simulink model "VehCtrlMdel240926_2018b_amkspdlimit"  (R2019b)
settings: Solver=FixedStepDiscrete  StartTime=0.0  StopTime=20  FixedStep=0.0005  RelTol=1e-3  EnableMultiTasking=on
undefined symbols (not defined in the file): Ax_OffSet, Ay_OffSet, Caf, Car, DiscIntNeverNeededParam, dwf, dwr, h, i1, i2, I_AN06_5V, I_AN07_5V, I_AN08_5V, I_AN09_5V, I_SW01_L, I_SW03_L, Iz, Kc, Ki, Kp, Ldwf, Ldwr, lf, lr, m, O_SW12_HS1A, O_SW14_HS1A, Offset_Angle, PWM3, Qa, Ra, Rt, thr1, thr2, thr3, thr4, thr5, TrqRquRate, YawRate_OffSet
libraries: simulink x150, ec5744lib x122, canmsglib x18
(part 4 of 5)

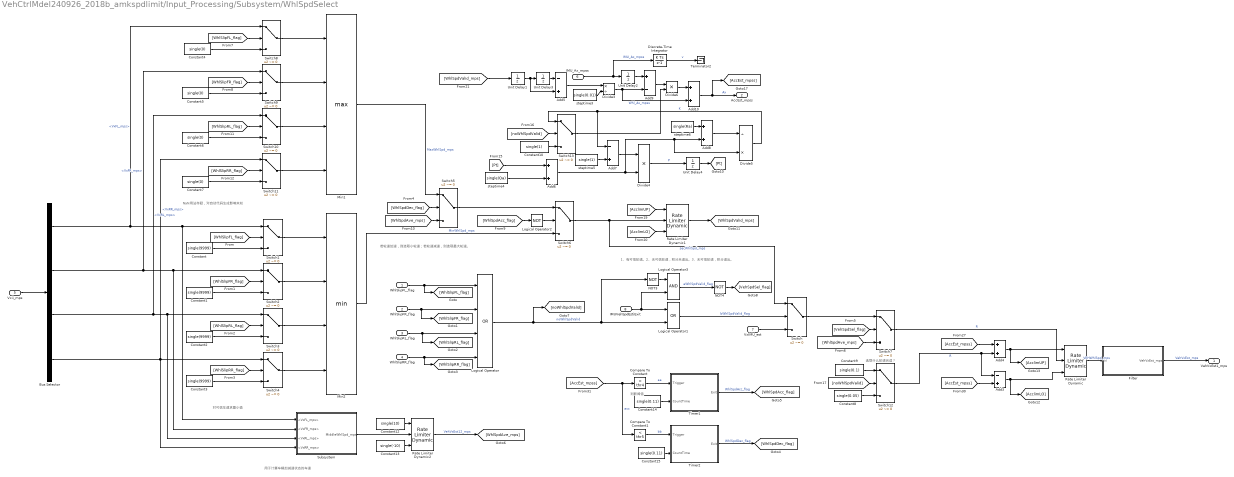
== system VehCtrlMdel240926_2018b_amkspdlimit/Input_Processing/Subsystem/WhlSpdSelect ==
  note: 用于计算车辆加减速状态的车速
  note: 1、有可信轮速。2、无可信轮速，积分未退出。3、无可信轮速，积分退出。
  note: 选取什么轮速合适？
  note: 判断阈值
  note: 若轮速加速，则选取小轮速；若轮速减速，则选取最大轮速。
  note: NaN用法存疑，对自动代码生成影响未知
  note: 对可信车速求最小值
  WhlSlipFL_flag : Inport
  WhlSlipFR_flag : Inport  Port=2
  WhlSlipRL_flag : Inport  Port=3
  WhlSlipRR_flag : Inport  Port=4
  Vxii_mps : Inport  Port=5
  IMU_Ax_mpss : Inport  Port=6
  VxIMU_est : Inport  Port=7
  IMUVehSpdEstiExit : Inport  Port=8
  Add{4,6,8,10} (4 alike) : Sum
  Add3 : Sum  Inputs=-+
  Add5 : Sum  Inputs=-+
  Add7 : Sum  Inputs=-+
  Add9 : Sum  Inputs=+-
  Bus Selector : BusSelector  OutputSignals=VxFL_mps,VxFR_mps,VxRL_mps,VxRR_mps
  Compare To Constant : simulink/Logic and Bit Operations/Compare To Constant  relop=>  const=thr4  OutDataTypeStr=boolean
  Compare To Constant1 : simulink/Logic and Bit Operations/Compare To Constant  relop=<  const=thr5  OutDataTypeStr=boolean
  Constant{,1..3} (4 alike) : Constant  Value=single(9999)
  Constant10 : Constant  Value=single(1)
  Constant12 : Constant  Value=single(10)
  Constant13 : Constant  Value=single(-10)
  Constant14 : Constant  Value=single(0.11)
  Constant15 : Constant  Value=single(0.11)
  Constant{4..7} (4 alike) : Constant  Value=single(0)
  Constant8 : Constant  Value=single(0.05)
  Constant9 : Constant  Value=single(0.1)
  Discrete-Time Integrator : DiscreteIntegrator  SampleTime=-1  ICPrevOutput=DiscIntNeverNeededParam  ICPrevScaledInput=DiscIntNeverNeededParam
  Divide3 : Product  Inputs=*/
  Divide4 : Product  Inputs=**
  Divide5 : Product  Inputs=/*
  Divide6 : Product  Inputs=**
  Filter : Subsystem
  Logical Operator : Logic  Operator=OR  Inputs=4  AllPortsSameDT=off  OutDataTypeStr=boolean
  Logical Operator1 : Logic  Operator=OR  AllPortsSameDT=off  OutDataTypeStr=boolean
  Logical Operator2 : Logic  Operator=NOT  AllPortsSameDT=off  OutDataTypeStr=boolean
  Logical Operator3 : Logic  AllPortsSameDT=off  OutDataTypeStr=boolean
  Min1 : MinMax  Function=max  Inputs=4
  Min2 : MinMax  Inputs=4
  NOT3 : Logic  Operator=NOT  AllPortsSameDT=off  OutDataTypeStr=boolean
  NOT4 : Logic  Operator=NOT  AllPortsSameDT=off  OutDataTypeStr=boolean
  Rate Limiter Dynamic : simulink/Discontinuities/Rate Limiter Dynamic
      settings: SourceProductName=Simulink
  Rate Limiter Dynamic1 : simulink/Discontinuities/Rate Limiter Dynamic
      settings: SourceProductName=Simulink
  Rate Limiter Dynamic2 : simulink/Discontinuities/Rate Limiter Dynamic
      settings: SourceProductName=Simulink
  Subsystem : Subsystem
  Switch{,1..13} (14 alike) : Switch  Criteria=u2 ~= 0
  Terminator2 : Terminator
  Timer1 : Stateflow chart  TreatAsAtomicUnit=on
  Timer2 : Stateflow chart  TreatAsAtomicUnit=on
  Unit Delay1 : UnitDelay  SampleTime=-1  HasFrameUpgradeWarning=on
  Unit Delay2 : UnitDelay  SampleTime=-1  HasFrameUpgradeWarning=on
  Unit Delay3 : UnitDelay  SampleTime=-1  HasFrameUpgradeWarning=on
  Unit Delay4 : UnitDelay  InitialCondition=0.01  SampleTime=-1  HasFrameUpgradeWarning=on
  steptime3 : Constant  Value=single(0.01)
  steptime4 : Constant  Value=single(Qa)
  steptime5 : Constant  Value=single(1)
  steptime6 : Constant  Value=single(Ra)
  VehVxEst1_mps : Outport
  AccEst_mpss : Outport  Port=2
  wires:
  Compare To Constant/1 -> Timer1/1(Trigger)  "aa"
  Vxii_mps/1 -> Bus Selector/1
  WhlSlipRR_flag/1 -> [WhlSlipRR_flag], Logical Operator/4
  Logical Operator3/1 -> NOT4/1  "aWhlSpdValid_flag"
  [VehSpdSel_flag] -> Switch7/2
  Logical Operator2/1 -> Switch6/2
  [WhlSlipFL_flag] -> Switch1/2
  Switch5/1 -> Switch6/1
  Constant/1 -> Switch1/3
  Compare To Constant1/1 -> Timer2/1(Trigger)  "bb"
  [WhlSpdAve_mps] -> Switch5/3
  Constant3/1 -> Switch4/3
  Logical Operator1/1 -> Switch/2  "bWhlSpdValid_flag"
  Switch4/1 -> Min2/4
  Constant2/1 -> Switch3/3
  [WhlSlipRR_flag] -> Switch4/2
  Switch1/1 -> Min2/1
  WhlSlipFR_flag/1 -> [WhlSlipFR_flag], Logical Operator/2
  [WhlSpdAcc_flag] -> Logical Operator2/1
  [WhlSlipRL_flag] -> Switch3/2
  Switch2/1 -> Min2/2
  WhlSlipFL_flag/1 -> [WhlSlipFL_flag], Logical Operator/1
  Constant1/1 -> Switch2/3
  [WhlSpdDec_flag] -> Switch5/2
  [WhlSlipFR_flag] -> Switch2/2
  WhlSlipRL_flag/1 -> [WhlSlipRL_flag], Logical Operator/3
  Switch3/1 -> Min2/3
  [WhlSpdAve_mps] -> Switch7/3
  Bus Selector/1 -> Switch8/1, Subsystem/1(<VxFL_mps>), Switch1/1  "<VxFL_mps>"
  Bus Selector/4 -> Subsystem/4(<VxRR_mps>), Switch11/1, Switch4/1  "<VxRR_mps>"
  [WhlSlipFR_flag] -> Switch9/2
  Bus Selector/2 -> Switch9/1, Subsystem/2(<VxFR_mps>), Switch2/1  "<VxFR_mps>"
  Constant5/1 -> Switch9/3
  Bus Selector/3 -> Switch10/1, Subsystem/3(<VxRL_mps>), Switch3/1  "<VxRL_mps>"
  [WhlSlipRL_flag] -> Switch10/2
  [WhlSlipRR_flag] -> Switch11/2
  Constant6/1 -> Switch10/3
  Constant7/1 -> Switch11/3
  Constant4/1 -> Switch8/3
  [WhlSlipFL_flag] -> Switch8/2
  Switch8/1 -> Min1/1
  Switch9/1 -> Min1/2
  Switch10/1 -> Min1/3
  Switch11/1 -> Min1/4
  Min1/1 -> Switch5/1  "MaxWhlSpd_mps"
  Subsystem/1(MiddleWhlSpd_mps) -> Rate Limiter Dynamic2/2
  Constant12/1 -> Rate Limiter Dynamic2/1
  Constant13/1 -> Rate Limiter Dynamic2/3
  Rate Limiter Dynamic2/1 -> [WhlSpdAve_mps]  "VehVxEst12_mps"
  Min2/1 -> Switch6/3  "MinWhlSpd_mps"
  IMUVehSpdEstiExit/1 -> Logical Operator3/2, Logical Operator1/1
  NOT3/1 -> Logical Operator3/1
  NOT4/1 -> [VehSpdSel_flag]
  Divide5/1 -> Add7/1, Switch13/1  "K"
  Unit Delay3/1 -> Add5/1
  steptime3/1 -> Divide3/2
  Add5/1 -> Divide3/1
  Unit Delay4/1 -> [Pt]
  [Pt] -> Add6/1
  steptime4/1 -> Add6/2
  Add6/1 -> Divide5/2, Add8/2, Divide4/2
  steptime5/1 -> Add7/2
  Add7/1 -> Divide4/1
  Divide4/1 -> Unit Delay4/1  "P"
  steptime6/1 -> Add8/1
  Add8/1 -> Divide5/1
  Divide3/1 -> Add10/2, Add9/2  "Whl_Ax_mpss"
  Add9/1 -> Divide6/1
  Divide6/1 -> Add10/1
  Add10/1 -> AccEst_mpss/1, [AccEst_mpss]  "Ax"
  IMU_Ax_mpss/1 -> Unit Delay2/1, Discrete-Time Integrator/1  "IMU_Ax_mpss"
  VxIMU_est/1 -> Switch/3
  Filter/1(VehVxEst_mps) -> VehVxEst1_mps/1  "VehVxEst_mps"
  Switch/1 -> Switch7/1
  Discrete-Time Integrator/1 -> Terminator2/1  "v"
  [AccEst_mpss] -> Add4/1
  [AccEst_mpss] -> Add3/2
  [WhlSpdValid_mps] -> Unit Delay1/1
  Unit Delay2/1 -> Add9/1
  Switch6/1 -> Switch/1, Rate Limiter Dynamic1/2  "secWhlSpd_mps"
  Add4/1 -> [AcclimUP], Rate Limiter Dynamic/1
  Add3/1 -> [AcclimLO], Rate Limiter Dynamic/3
  Switch7/1 -> Rate Limiter Dynamic/2  "R"
  Rate Limiter Dynamic/1 -> Filter/1(In)  "VEHWhlSpd_mps"
  Rate Limiter Dynamic1/1 -> [WhlSpdValid_mps]
  Unit Delay1/1 -> Add5/2, Unit Delay3/1
  [noWhlSpdValid] -> Switch12/2
  Constant8/1 -> Switch12/3
  Constant9/1 -> Switch12/1
  Switch12/1 -> Add3/1, Add4/2  "R"
  Switch13/1 -> Divide6/2
  [noWhlSpdValid] -> Switch13/2
  Constant10/1 -> Switch13/3
  [AcclimUP] -> Rate Limiter Dynamic1/1
  [AcclimLO] -> Rate Limiter Dynamic1/3
  Logical Operator/1 -> NOT3/1, Logical Operator1/2, [noWhlSpdValid]  "noWhlSpdValid"
  Timer1/1(Exit) -> [WhlSpdAcc_flag]  "WhlSpdAcc_flag"
  Constant14/1 -> Timer1/2(CountTime)
  Timer2/1(Exit) -> [WhlSpdDec_flag]  "WhlSpdDec_flag"
  Constant15/1 -> Timer2/2(CountTime)
  [AccEst_mpss] -> Compare To Constant1/1, Compare To Constant/1  "acc"

== system VehCtrlMdel240926_2018b_amkspdlimit/Input_Processing/Subsystem/坐标系转换 ==
  note: cos模块的单位是弧度制、
  note: 未考虑漂移工况
  note: 顺时针为正，逆时针为负。
  WhlSpdFL_mps : Inport
  WhlSpdFR_mps : Inport  Port=2
  WhlSpdRL_mps : Inport  Port=3
  WhlSpdRR_mps : Inport  Port=4
  IMU_YawRate_dps : Inport  Port=5
  WhlStrAngL_deg : Inport  Port=6
  WhlStrAngR_deg : Inport  Port=7
  Add : Sum  Inputs=+-
  Add1 : Sum
  Add2 : Sum  Inputs=+-
  Add3 : Sum
  Asin : Trigonometry  Operator=cos
  Asin1 : Trigonometry  Operator=cos
  Bus Creator : BusCreator  Inputs=4
  Constant : Constant  Value=single(Ldwr)
  Constant1 : Constant  Value=single(Ldwf)
  Gain : Gain  Gain=1/2
  Gain1 : Gain  Gain=1/2
  Gain2 : Gain  Gain=pi/180
  Gain3 : Gain  Gain=pi/180
  Gain4 : Gain  Gain=pi/180
  Product{,1..3} (4 alike) : Product
  Vxii_mps : Outport
  IMU_YawRate_dps1 : Outport  Port=2
  wires:
  Constant/1 -> Gain/1
  Gain/1 -> Product/2
  IMU_YawRate_dps/1 -> Gain4/1  "IMU_YawRate_dps"
  WhlSpdRL_mps/1 -> Add/1  "WhlSpdRL_mps"
  WhlSpdRR_mps/1 -> Add1/2  "WhlSpdRR_mps"
  Product/1 -> [Vldwr]
  [Vldwr] -> Add/2, Add1/1
  WhlSpdFL_mps/1 -> Product1/1  "WhlSpdFL_mps"
  WhlSpdFR_mps/1 -> Product2/2  "WhlSpdFR_mps"
  Constant1/1 -> Gain1/1
  Gain1/1 -> Product3/1
  Product3/1 -> [Vldwf]
  Product1/1 -> Add2/1  "1"
  [Vldwf] -> Add2/2, Add3/1  "3"
  Product2/1 -> Add3/2
  Add2/1 -> Bus Creator/1  "VxFL_mps"
  Add/1 -> Bus Creator/3  "VxRL_mps"
  Add3/1 -> Bus Creator/2  "VxFR_mps"
  Add1/1 -> Bus Creator/4  "VxRR_mps"
  Bus Creator/1 -> Vxii_mps/1
  Asin1/1 -> Product2/1
  WhlStrAngR_deg/1 -> Gain3/1  "WhlStrAngR_deg"
  WhlStrAngL_deg/1 -> Gain2/1  "WhlStrAngL_deg"
  Asin/1 -> Product1/2  "a"
  Gain2/1 -> Asin/1
  Gain3/1 -> Asin1/1
  Gain4/1 -> IMU_YawRate_dps1/1, Product/1, Product3/2

== system VehCtrlMdel240926_2018b_amkspdlimit/CTRL/MoTrqReq/TCS_PI+FF_Ctrl_FL/Latch_on ==
  Set : Inport
  Reset : Inport  Port=2
  Logical Operator4 : Logic  Operator=NOR  AllPortsSameDT=off  OutDataTypeStr=boolean
  Logical Operator5 : Logic  Operator=NOR  AllPortsSameDT=off  OutDataTypeStr=boolean
  Unit Delay1 : UnitDelay  SampleTime=-1  HasFrameUpgradeWarning=on
  flg_TCSActv : Outport
  wires:
  Logical Operator5/1 -> flg_TCSActv/1, Unit Delay1/1
  Reset/1 -> Logical Operator5/2
  Unit Delay1/1 -> Logical Operator4/1
  Set/1 -> Logical Operator4/2
  Logical Operator4/1 -> Logical Operator5/1

== system VehCtrlMdel240926_2018b_amkspdlimit/CTRL/MoTrqReq/TCS_PI+FF_Ctrl_FL/RisingTimer ==
  Set : Inport
  Timer : Inport  Port=2
  Add10 : Sum
  Min : MinMax  Inputs=2
  Relational Operator9 : RelationalOperator  OutDataTypeStr=boolean  RndMeth=Simplest
  Reset : Constant  Value=single(0)
  Steptime : Constant  Value=single(0.01)
  Switch6 : Switch  Criteria=u2 ~= 0
  Unit Delay1 : UnitDelay  SampleTime=-1  HasFrameUpgradeWarning=on
  TCSExit : Outport
  wires:
  Add10/1 -> Switch6/1
  Set/1 -> Switch6/2
  Min/1 -> Unit Delay1/1, Relational Operator9/1
  Unit Delay1/1 -> Add10/1
  Timer/1 -> Relational Operator9/2, Min/2
  Reset/1 -> Switch6/3
  Relational Operator9/1 -> TCSExit/1
  Steptime/1 -> Add10/2
  Switch6/1 -> Min/1

== system VehCtrlMdel240926_2018b_amkspdlimit/CTRL/MoTrqReq/TCS_PI+FF_Ctrl_FR/Latch_on ==
  Set : Inport
  Reset : Inport  Port=2
  Logical Operator4 : Logic  Operator=NOR  AllPortsSameDT=off  OutDataTypeStr=boolean
  Logical Operator5 : Logic  Operator=NOR  AllPortsSameDT=off  OutDataTypeStr=boolean
  Unit Delay1 : UnitDelay  SampleTime=-1  HasFrameUpgradeWarning=on
  flg_TCSActv : Outport
  wires:
  Logical Operator4/1 -> Logical Operator5/1
  Set/1 -> Logical Operator4/2
  Unit Delay1/1 -> Logical Operator4/1
  Reset/1 -> Logical Operator5/2
  Logical Operator5/1 -> Unit Delay1/1, flg_TCSActv/1

== system VehCtrlMdel240926_2018b_amkspdlimit/CTRL/MoTrqReq/TCS_PI+FF_Ctrl_FR/RisingTimer ==
  Set : Inport
  Timer : Inport  Port=2
  Add10 : Sum
  Min : MinMax  Inputs=2
  Relational Operator9 : RelationalOperator  OutDataTypeStr=boolean  RndMeth=Simplest
  Reset : Constant  Value=single(0)
  Steptime : Constant  Value=single(0.01)
  Switch6 : Switch  Criteria=u2 ~= 0
  Unit Delay1 : UnitDelay  SampleTime=-1  HasFrameUpgradeWarning=on
  TCSExit : Outport
  wires:
  Switch6/1 -> Min/1
  Steptime/1 -> Add10/2
  Relational Operator9/1 -> TCSExit/1
  Reset/1 -> Switch6/3
  Timer/1 -> Min/2, Relational Operator9/2
  Unit Delay1/1 -> Add10/1
  Min/1 -> Relational Operator9/1, Unit Delay1/1
  Set/1 -> Switch6/2
  Add10/1 -> Switch6/1

== system VehCtrlMdel240926_2018b_amkspdlimit/CTRL/MoTrqReq/TCS_PI+FF_Ctrl_R/Latch_on ==
  Set : Inport
  Reset : Inport  Port=2
  Logical Operator4 : Logic  Operator=NOR  AllPortsSameDT=off  OutDataTypeStr=boolean
  Logical Operator5 : Logic  Operator=NOR  AllPortsSameDT=off  OutDataTypeStr=boolean
  Unit Delay1 : UnitDelay  SampleTime=-1  HasFrameUpgradeWarning=on
  flg_TCSActv : Outport
  wires:
  Logical Operator5/1 -> flg_TCSActv/1, Unit Delay1/1
  Reset/1 -> Logical Operator5/2
  Unit Delay1/1 -> Logical Operator4/1
  Set/1 -> Logical Operator4/2
  Logical Operator4/1 -> Logical Operator5/1

== system VehCtrlMdel240926_2018b_amkspdlimit/CTRL/MoTrqReq/TCS_PI+FF_Ctrl_R/RisingTimer ==
  Set : Inport
  Timer : Inport  Port=2
  Add10 : Sum
  Min : MinMax  Inputs=2
  Relational Operator9 : RelationalOperator  OutDataTypeStr=boolean  RndMeth=Simplest
  Reset : Constant  Value=single(0)
  Steptime : Constant  Value=single(0.01)
  Switch6 : Switch  Criteria=u2 ~= 0
  Unit Delay1 : UnitDelay  SampleTime=-1  HasFrameUpgradeWarning=on
  TCSExit : Outport
  wires:
  Add10/1 -> Switch6/1
  Set/1 -> Switch6/2
  Min/1 -> Unit Delay1/1, Relational Operator9/1
  Unit Delay1/1 -> Add10/1
  Timer/1 -> Relational Operator9/2, Min/2
  Reset/1 -> Switch6/3
  Relational Operator9/1 -> TCSExit/1
  Steptime/1 -> Add10/2
  Switch6/1 -> Min/1

== system VehCtrlMdel240926_2018b_amkspdlimit/Input/ABS_Receive/ABS_BUS_state/IMU_state ==
  ID : Inport
  Msg : Inport  Port=2
  Enable : EnablePort
  CAN Unpack1 : canmsglib/CAN Unpack  CANdbFile=d:\Users\YJR\Desktop\DBC\Abs_Dev_Dbc_20240603_NingYuan.dbc  MsgList=ABS_Basic_Msg2  MsgName=ABS_Basic_Msg2  MsgIDType=Standard (11-bit identifier)  MsgIdentifier=1698  MsgLength=8  SignalInfo={'WS_FL','8','16','BE','signed','Standard','0','0.014063','0','-460.8','460.7859';'WS_FR','24','16','BE','signed','Standard','0','0.014063','0','-460.8','460.7859';'WS_RL','40','16','BE','signed','Standard','0','0.014063','0','-460.8','460.7859';'WS_RR','56','16','BE','signed','Standard','0','0.014063','0','-460.8','460.7859'}  IDPort=off  TimestampPort=off  ErrorPort=off  RemotePort=off  LengthPort=off  StatusPort=off  ApplyMinMax=off
      settings: SourceProductName=Simulink Real-Time  SourceProductBaseCode=XP  DataFormat=CANdb specified signals
  CANUnPackMessage4 : ec5744lib/RapidECU_U3/04CANCommunication/CANUnPackMessage  datalength=8  canmessagetype=Standard(11-bit ID)  sampletime=-1
      settings: SourceProductName=ECUCoder for MPC5744
  MeaModule1 : ec5744lib/RapidECU_U3/07Calibration/MeaModule  signal=ABS_WS_FR
      settings: SourceProductName=ECUCoder for MPC5744
  MeaModule2 : ec5744lib/RapidECU_U3/07Calibration/MeaModule  signal=ABS_WS_RL
      settings: SourceProductName=ECUCoder for MPC5744
  MeaModule3 : ec5744lib/RapidECU_U3/07Calibration/MeaModule  signal=ABS_WS_FL
      settings: SourceProductName=ECUCoder for MPC5744
  MeaModule4 : ec5744lib/RapidECU_U3/07Calibration/MeaModule  signal=ABS_WS_RR
      settings: SourceProductName=ECUCoder for MPC5744
  ABS_WS_FR : Outport  VectorParamsAs1DForOutWhenUnconnected=off
  ABS_WS_RL : Outport  Port=2  VectorParamsAs1DForOutWhenUnconnected=off
  ABS_WS_FL : Outport  Port=3  VectorParamsAs1DForOutWhenUnconnected=off
  ABS_WS_RR : Outport  Port=4  VectorParamsAs1DForOutWhenUnconnected=off
  wires:
  CAN Unpack1/3 -> MeaModule2/1  "ABS_WS_RL"
  CAN Unpack1/2 -> MeaModule1/1  "ABS_WS_FR"
  CAN Unpack1/1 -> MeaModule3/1  "ABS_WS_FL"
  CANUnPackMessage4/1 -> CAN Unpack1/1
  ID/1 -> CANUnPackMessage4/1
  Msg/1 -> CANUnPackMessage4/2
  CAN Unpack1/4 -> MeaModule4/1  "ABS_WS_RR"
  MeaModule3/1 -> ABS_WS_FL/1
  MeaModule1/1 -> ABS_WS_FR/1
  MeaModule2/1 -> ABS_WS_RL/1
  MeaModule4/1 -> ABS_WS_RR/1

== system VehCtrlMdel240926_2018b_amkspdlimit/Input/AMKMCU_Receive/FLAMKMCU/AMKMCU_state ==
  CANOK : Inport
  ID : Inport  Port=2
  Msg : Inport  Port=3
  function : TriggerPort  TriggerType=function-call  VariantControl=(inherit)
  MCU_state : Subsystem  TreatAsAtomicUnit=on
  FLAMKtoVCU1 : Outport  VectorParamsAs1DForOutWhenUnconnected=off
  wires:
  Msg/1 -> MCU_state/2(Msg)
  CANOK/1 -> MCU_state/Enable
  ID/1 -> MCU_state/1(ID)
  MCU_state/1(FLAMKMCUtoVCU1) -> FLAMKtoVCU1/1

== system VehCtrlMdel240926_2018b_amkspdlimit/Input/AMKMCU_Receive/FLAMKMCU/AMKMCU_state1 ==
  CANOK : Inport
  ID : Inport  Port=2
  Msg : Inport  Port=3
  function : TriggerPort  TriggerType=function-call  VariantControl=(inherit)
  Bus Creator : BusCreator  Inputs=2
  MCU_state : Subsystem  TreatAsAtomicUnit=on
  FLAMKMCUtoVCU2 : Outport  VectorParamsAs1DForOutWhenUnconnected=off
  wires:
  MCU_state/2(MCFL_ErrorInfo) -> Bus Creator/2
  MCU_state/1(MCFL_DiagnosticNum) -> Bus Creator/1
  Bus Creator/1 -> FLAMKMCUtoVCU2/1
  ID/1 -> MCU_state/1(ID)
  CANOK/1 -> MCU_state/Enable
  Msg/1 -> MCU_state/2(Msg)

== system VehCtrlMdel240926_2018b_amkspdlimit/Input/AMKMCU_Receive/FLAMKMCU/AMKMCU_state2 ==
  CANOK : Inport
  ID : Inport  Port=2
  Msg : Inport  Port=3
  function : TriggerPort  TriggerType=function-call  VariantControl=(inherit)
  Bus Creator : BusCreator  Inputs=3
  MCU_state : Subsystem  TreatAsAtomicUnit=on
  FLAMKMCUtoVCU3 : Outport  VectorParamsAs1DForOutWhenUnconnected=off
  wires:
  Msg/1 -> MCU_state/2(Msg)
  CANOK/1 -> MCU_state/Enable
  ID/1 -> MCU_state/1(ID)
  Bus Creator/1 -> FLAMKMCUtoVCU3/1  "Bus Creator"
  MCU_state/1(MCFL_TempIGBT) -> Bus Creator/1
  MCU_state/2(MCFL_TempInverter) -> Bus Creator/2
  MCU_state/3(MCFL_TempMotor) -> Bus Creator/3

== system VehCtrlMdel240926_2018b_amkspdlimit/Input/AMKMCU_Receive/FRAMKMCU/AMKMCU_state ==
  CANOK : Inport
  ID : Inport  Port=2
  Msg : Inport  Port=3
  function : TriggerPort  TriggerType=function-call  VariantControl=(inherit)
  Bus Creator : BusCreator  Inputs=12
  MCU_state : Subsystem  TreatAsAtomicUnit=on
  FRAMKMCUtoVCU1 : Outport  VectorParamsAs1DForOutWhenUnconnected=off
  wires:
  ID/1 -> MCU_state/1(ID)
  CANOK/1 -> MCU_state/Enable
  Msg/1 -> MCU_state/2(Msg)
  MCU_state/1(MCFR_ActualTorque) -> Bus Creator/1
  MCU_state/2(MCFR_ActualVelocity) -> Bus Creator/2
  MCU_state/3(MCFR_DCVoltage) -> Bus Creator/3
  MCU_state/4(MCFR_bDCOn) -> Bus Creator/4
  MCU_state/5(MCFR_bDerating) -> Bus Creator/5
  MCU_state/6(MCFR_bError) -> Bus Creator/6
  MCU_state/7(MCFR_bInverterOn) -> Bus Creator/7
  MCU_state/8(MCFR_bQuitDCOn) -> Bus Creator/8
  MCU_state/9(MCFR_bQuitInverterOn) -> Bus Creator/9
  MCU_state/10(MCFR_bReserve) -> Bus Creator/10
  MCU_state/11(MCFR_bSystemReady) -> Bus Creator/11
  MCU_state/12(MCFR_bWarn) -> Bus Creator/12
  Bus Creator/1 -> FRAMKMCUtoVCU1/1

== system VehCtrlMdel240926_2018b_amkspdlimit/Input/AMKMCU_Receive/FRAMKMCU/AMKMCU_state1 ==
  CANOK : Inport
  ID : Inport  Port=2
  Msg : Inport  Port=3
  function : TriggerPort  TriggerType=function-call  VariantControl=(inherit)
  Bus Creator : BusCreator  Inputs=2
  MCU_state : Subsystem  TreatAsAtomicUnit=on
  FRAMKMCUtoVCU2 : Outport  VectorParamsAs1DForOutWhenUnconnected=off
  wires:
  Msg/1 -> MCU_state/2(Msg)
  CANOK/1 -> MCU_state/Enable
  ID/1 -> MCU_state/1(ID)
  Bus Creator/1 -> FRAMKMCUtoVCU2/1
  MCU_state/1(MCFR_DiagnosticNum) -> Bus Creator/1
  MCU_state/2(MCFR_ErrorInfo) -> Bus Creator/2

== system VehCtrlMdel240926_2018b_amkspdlimit/Input/AMKMCU_Receive/FRAMKMCU/AMKMCU_state2 ==
  CANOK : Inport
  ID : Inport  Port=2
  Msg : Inport  Port=3
  function : TriggerPort  TriggerType=function-call  VariantControl=(inherit)
  Bus Creator : BusCreator  Inputs=3
  MCU_state : Subsystem  TreatAsAtomicUnit=on
  FRAMKMCUtoVCU3 : Outport  VectorParamsAs1DForOutWhenUnconnected=off
  wires:
  Bus Creator/1 -> FRAMKMCUtoVCU3/1
  ID/1 -> MCU_state/1(ID)
  CANOK/1 -> MCU_state/Enable
  Msg/1 -> MCU_state/2(Msg)
  MCU_state/1(MCFR_TempIGBT) -> Bus Creator/1
  MCU_state/2(MCFR_TempInverter) -> Bus Creator/2
  MCU_state/3(MCFR_TempMotor) -> Bus Creator/3

== system VehCtrlMdel240926_2018b_amkspdlimit/Input/BMS_Recive/ABS_BUS_state/IMU_state ==
  ID : Inport
  Msg : Inport  Port=2
  Enable : EnablePort
  CAN Unpack1 : canmsglib/CAN Unpack  CANdbFile=d:\Users\YJR\Desktop\DBC\bms.dbc  MsgList=BMS_HCU_INFO  MsgName=BMS_HCU_INFO  MsgIDType=Extended (29-bit identifier)  MsgIdentifier=408961267  MsgLength=8  SignalInfo={'BatAlmlv','52','4','LE','signed','Standard','0','1','0','0','4';'BatLife','56','8','LE','signed','Standard','0','1','0','0','255';'BatState','48','4','LE','signed','Standard','0','1','0','0','7';'LSBAz','24','8','LE','signed','Standard','0','0.1','-1000','-1012.8','-987.3';'LSBVz','8','8','LE','unsigned','Standard','0','0.1','0','0','9000';'MSBAz','16','8','LE','unsigned','Standard','0','0.1','-1000','-1000','-974.5';'MSBVz','0','8','LE','unsigned','Standard','0','0.1','0','0','9000';'SOCz','32','8','LE','signed','Standard','0','1','0','0','100';'SOHz','40','8','LE','signed','Standard','0','1','0','0','100'}  IDPort=off  TimestampPort=off  ErrorPort=off  RemotePort=off  LengthPort=off  StatusPort=off  ApplyMinMax=off
      settings: SourceProductName=Simulink Real-Time  SourceProductBaseCode=XP  DataFormat=CANdb specified signals
  CANUnPackMessage4 : ec5744lib/RapidECU_U3/04CANCommunication/CANUnPackMessage  datalength=8  canmessagetype=Extended(29-bit ID)  sampletime=-1
      settings: SourceProductName=ECUCoder for MPC5744
  BatAlmlv : Outport  VectorParamsAs1DForOutWhenUnconnected=off
  BatLife : Outport  Port=2  VectorParamsAs1DForOutWhenUnconnected=off
  BatState : Outport  Port=3  VectorParamsAs1DForOutWhenUnconnected=off
  LSBAz : Outport  Port=4  VectorParamsAs1DForOutWhenUnconnected=off
  LSBVz : Outport  Port=5  VectorParamsAs1DForOutWhenUnconnected=off
  MSBAz : Outport  Port=6  VectorParamsAs1DForOutWhenUnconnected=off
  MSBVz : Outport  Port=7  VectorParamsAs1DForOutWhenUnconnected=off
  SOCz : Outport  Port=8  VectorParamsAs1DForOutWhenUnconnected=off
  SOHz : Outport  Port=9  VectorParamsAs1DForOutWhenUnconnected=off
  wires:
  CANUnPackMessage4/1 -> CAN Unpack1/1
  ID/1 -> CANUnPackMessage4/1
  Msg/1 -> CANUnPackMessage4/2
  CAN Unpack1/1 -> BatAlmlv/1  "BatAlmlv"
  CAN Unpack1/2 -> BatLife/1  "BatLife"
  CAN Unpack1/3 -> BatState/1  "BatState"
  CAN Unpack1/4 -> LSBAz/1  "LSBAz"
  CAN Unpack1/5 -> LSBVz/1  "LSBVz"
  CAN Unpack1/6 -> MSBAz/1  "MSBAz"
  CAN Unpack1/7 -> MSBVz/1  "MSBVz"
  CAN Unpack1/8 -> SOCz/1  "SOCz"
  CAN Unpack1/9 -> SOHz/1  "SOHz"

== system VehCtrlMdel240926_2018b_amkspdlimit/Input/EMRAXMCU_RECIEVE/MCU_pwr/MCU_VCUMeter1 ==
  ID : Inport
  Msg : Inport  Port=2
  Enable : EnablePort
  CAN Unpack : canmsglib/CAN Unpack  CANdbFile=E:\candbc\MCU_No1.dbc  MsgList=(none)  MsgName=MCU2VCU2_ID1  MsgIDType=Extended (29-bit identifier)  MsgIdentifier=218089455  MsgLength=8  SignalInfo={'MCU2VCU2_Current_AC_Feedback_ID1','48','16','LE','unsigned','Standard','0','1.000000e-01','-1600','-1600','1600';'MCU2VCU2_Current_DC_feedback_ID1','32','16','LE','unsigned','Standard','0','1.000000e-01','-1600','-1600','1600';'MCU2VCU2_MCU_Temp_ID1','0','8','LE','unsigned','Standard','0','1','-50','-50','200';'MCU2VCU2_Motor_Temp_ID1','8','8','LE','unsigned','Standard','0','1','-50','-50','200';'MCU2VCU2_Voltage_Feedback_ID1','16','16','LE','unsigned','Standard','0','1.000000e-01','0','0','1000'}  IDPort=off  TimestampPort=off  ErrorPort=off  RemotePort=off  LengthPort=off  StatusPort=off  ApplyMinMax=off
      settings: SourceProductName=Vehicle Network Toolbox  SourceProductBaseCode=VN  DataFormat=CANdb specified signals
  CANUnPackMessage4 : ec5744lib/RapidECU_U3/04CANCommunication/CANUnPackMessage  datalength=8  canmessagetype=Extended(29-bit ID)  sampletime=-1
      settings: SourceProductName=ECUCoder for MPC5744
  MeaModule1 : ec5744lib/RapidECU_U3/07Calibration/MeaModule  signal=AC_current
      settings: SourceProductName=ECUCoder for MPC5744
  MeaModule2 : ec5744lib/RapidECU_U3/07Calibration/MeaModule  signal=DC_current
      settings: SourceProductName=ECUCoder for MPC5744
  MeaModule3 : ec5744lib/RapidECU_U3/07Calibration/MeaModule  signal=MCU_Temp
      settings: SourceProductName=ECUCoder for MPC5744
  MeaModule4 : ec5744lib/RapidECU_U3/07Calibration/MeaModule  signal=motor_Temp
      settings: SourceProductName=ECUCoder for MPC5744
  MeaModule5 : ec5744lib/RapidECU_U3/07Calibration/MeaModule  signal=voltage
      settings: SourceProductName=ECUCoder for MPC5744
  "AC_current " : Outport
  MCU_temp : Outport  Port=2
  current : Outport  Port=3
  motor_temp : Outport  Port=4
  voltage : Outport  Port=5
  wires:
  Msg/1 -> CANUnPackMessage4/2
  ID/1 -> CANUnPackMessage4/1
  CANUnPackMessage4/1 -> CAN Unpack/1
  CAN Unpack/1 -> MeaModule1/1  "AC_current"
  CAN Unpack/5 -> MeaModule5/1  "voltage"
  CAN Unpack/4 -> MeaModule4/1  "moter_temp"
  MeaModule1/1 -> "AC_current "/1
  MeaModule2/1 -> current/1
  CAN Unpack/3 -> MeaModule3/1  "MCU_temp"
  CAN Unpack/2 -> MeaModule2/1  "DC_current"
  MeaModule3/1 -> MCU_temp/1
  MeaModule4/1 -> motor_temp/1
  MeaModule5/1 -> voltage/1

== system VehCtrlMdel240926_2018b_amkspdlimit/Input/EMRAXMCU_RECIEVE/MCU_state/MCU_state ==
  ID : Inport
  Msg : Inport  Port=2
  Enable : EnablePort
  CAN Unpack : canmsglib/CAN Unpack  CANdbFile=E:\candbc\MCU_No1.dbc  MsgList=(none)  MsgName=MCU2VCU1_ID1  MsgIDType=Extended (29-bit identifier)  MsgIdentifier=218089199  MsgLength=8  SignalInfo={'MCU2VCU1_12V_error_ID1','45','1','LE','unsigned','Standard','0','1','0','0','1';'MCU2VCU1_Error_All_ID1','56','2','LE','unsigned','Standard','0','1','0','0','3';'MCU2VCU1_LowVoltage_error_ID1','46','1','LE','unsigned','Standard','0','1','0','0','1';'MCU2VCU1_MCU_Ready_ID1','40','1','LE','unsigned','Standard','0','1','0','0','1';'MCU2VCU1_MCU_Temp_error_ID1','48','1','LE','unsigned','Standard','0','1','0','0','1';'MCU2VCU1_Mode_Feedback_ID1','32','8','LE','unsigned','Standard','0','1','0','0','255';'MCU2VCU1_MotorTemp_error_ID1','49','1','LE','unsigned','Standard','0','1','0','0','1';'MCU2VCU1_OverCurrent_error_ID1','43','1','LE','unsigned','Standard','0','1','0','0','1';'MCU2VCU1_OverPower_error_ID1','47','1','LE','unsigned','Standard','0','1','0','0','1';'MCU2VCU1_OverVoltage_error_ID1','44','1','LE','unsigned','Standard','0','1','0','0','1';'MCU2VCU1_PrechargeState_ID1','41','1','LE','unsigned','Standard','0','1','0','0','1';'MCU2VCU1_Reslove_Error_ID1','42','1','LE','unsigned','Standard','0','1','0','0','1';'MCU2VCU1_Selfcheck_ID1','55','1','LE','unsigned','Standard','0','1','0','0','1';'MCU2VCU1_Speed_Feedback_ID1','0','16','LE','unsigned','Standard','0','5.000000e-01','-10000','-10000','10000';'MCU2VCU1_Torque_Feedback_ID1','16','16','LE','unsigned','Standard','0','1','0','0','1000'}  IDPort=off  TimestampPort=off  ErrorPort=off  RemotePort=off  LengthPort=off  StatusPort=off  ApplyMinMax=off
      settings: SourceProductName=Vehicle Network Toolbox  SourceProductBaseCode=VN  DataFormat=CANdb specified signals
  CANUnPackMessage4 : ec5744lib/RapidECU_U3/04CANCommunication/CANUnPackMessage  datalength=8  canmessagetype=Extended(29-bit ID)  sampletime=-1
      settings: SourceProductName=ECUCoder for MPC5744
  MeaModule : ec5744lib/RapidECU_U3/07Calibration/MeaModule  signal=RPM
      settings: SourceProductName=ECUCoder for MPC5744
  MeaModule1 : ec5744lib/RapidECU_U3/07Calibration/MeaModule  signal=alarm
      settings: SourceProductName=ECUCoder for MPC5744
  MeaModule2 : ec5744lib/RapidECU_U3/07Calibration/MeaModule  signal=L12V_error
      settings: SourceProductName=ECUCoder for MPC5744
  MeaModule3 : ec5744lib/RapidECU_U3/07Calibration/MeaModule  signal=controller_ready
      settings: SourceProductName=ECUCoder for MPC5744
  MeaModule5 : ec5744lib/RapidECU_U3/07Calibration/MeaModule  signal=selfcheck
      settings: SourceProductName=ECUCoder for MPC5744
  MeaModule6 : ec5744lib/RapidECU_U3/07Calibration/MeaModule  signal=trq
      settings: SourceProductName=ECUCoder for MPC5744
  12V_error : Outport
  alarm : Outport  Port=2
  undervol : Outport  Port=3
  controller_ready : Outport  Port=4
  MCU_temp_warn : Outport  Port=5
  mode_cmd8 : Outport  Port=6
  motor_temp_warn : Outport  Port=7
  overcur : Outport  Port=8
  pow_lim_warn : Outport  Port=9
  overvol : Outport  Port=10
  precharge : Outport  Port=11
  rotation_warn : Outport  Port=12
  selfcech : Outport  Port=13
  RPM : Outport  Port=14
  torque : Outport  Port=15
  wires:
  Msg/1 -> CANUnPackMessage4/2
  ID/1 -> CANUnPackMessage4/1
  CANUnPackMessage4/1 -> CAN Unpack/1
  MeaModule/1 -> RPM/1  "RPM"
  MeaModule1/1 -> alarm/1
  MeaModule2/1 -> 12V_error/1
  MeaModule3/1 -> controller_ready/1
  MeaModule5/1 -> selfcech/1
  MeaModule6/1 -> torque/1  "Trq"
  CAN Unpack/14 -> MeaModule/1  "RPM"
  CAN Unpack/15 -> MeaModule6/1  "Trq"
  CAN Unpack/13 -> MeaModule5/1
  CAN Unpack/11 -> precharge/1  "Precharge"
  CAN Unpack/10 -> overvol/1  "overvol"
  CAN Unpack/9 -> pow_lim_warn/1  "overpower"
  CAN Unpack/8 -> overcur/1  "overCurrent"
  CAN Unpack/7 -> motor_temp_warn/1  "motorTemp_error"
  CAN Unpack/6 -> mode_cmd8/1  "Mode"
  CAN Unpack/5 -> MCU_temp_warn/1  "MCU_Temp_error"
  CAN Unpack/4 -> MeaModule3/1  "MCU_Ready"
  CAN Unpack/3 -> undervol/1  "low_VOL"
  CAN Unpack/2 -> MeaModule1/1  "Error_ALL"
  CAN Unpack/1 -> MeaModule2/1  "12V_error"
  CAN Unpack/12 -> rotation_warn/1  "Reslove_error"

== system VehCtrlMdel240926_2018b_amkspdlimit/Input/IMU_Recieve/IMU_state/MCU_state ==
  ID : Inport
  Msg : Inport  Port=2
  Enable : EnablePort
  CAN Unpack : canmsglib/CAN Unpack  CANdbFile=d:\Users\YJR\Desktop\IMU.dbc  MsgList=(none)  MsgName=IMU  MsgIDType=Standard (11-bit identifier)  MsgIdentifier=513  MsgLength=8  SignalInfo={'IMU_Ax_Valid','1','1','LE','unsigned','Standard','0','1','0','-Inf','Inf';'IMU_Ax_Value','40','16','LE','unsigned','Standard','0','1.500000e-04','-4.915200e+00','-Inf','Inf';'IMU_Ay_Valid','2','1','LE','unsigned','Standard','0','1','0','-Inf','Inf';'IMU_Ay_Value','24','16','LE','unsigned','Standard','0','1.500000e-04','-4.915200e+00','-Inf','Inf';'IMU_DTC','4','4','LE','unsigned','Standard','0','1','0','-Inf','Inf';'IMU_Yaw_Valid','3','1','LE','unsigned','Standard','0','1','0','-Inf','Inf';'IMU_Yaw_Value','8','16','LE','unsigned','Standard','0','5.710000e-03','-1.872400e+02','-Inf','Inf'}  IDPort=off  TimestampPort=off  ErrorPort=off  RemotePort=off  LengthPort=off  StatusPort=off  ApplyMinMax=off
      settings: SourceProductName=Simulink Real-Time  SourceProductBaseCode=XP  DataFormat=CANdb specified signals
  CANUnPackMessage4 : ec5744lib/RapidECU_U3/04CANCommunication/CANUnPackMessage  datalength=8  canmessagetype=Standard(11-bit ID)  sampletime=-1
      settings: SourceProductName=ECUCoder for MPC5744
  MeaModule2 : ec5744lib/RapidECU_U3/07Calibration/MeaModule  signal=IMU_Ay_Value
      settings: SourceProductName=ECUCoder for MPC5744
  MeaModule3 : ec5744lib/RapidECU_U3/07Calibration/MeaModule  signal=IMU_Yaw_Value
      settings: SourceProductName=ECUCoder for MPC5744
  MeaModule4 : ec5744lib/RapidECU_U3/07Calibration/MeaModule  signal=IMU_Ax_Value
      settings: SourceProductName=ECUCoder for MPC5744
  IMU_Ax_Value : Outport  VectorParamsAs1DForOutWhenUnconnected=off
  IMU_Ay_Value : Outport  Port=2  VectorParamsAs1DForOutWhenUnconnected=off
  IMU_Yaw_Value : Outport  Port=3  VectorParamsAs1DForOutWhenUnconnected=off
  IMU_Ay_Valid : Outport  Port=4  VectorParamsAs1DForOutWhenUnconnected=off
  IMU_DTC : Outport  Port=5  VectorParamsAs1DForOutWhenUnconnected=off
  IMU_Yaw_Valid : Outport  Port=6  VectorParamsAs1DForOutWhenUnconnected=off
  IMU_Ax_Valid : Outport  Port=7  VectorParamsAs1DForOutWhenUnconnected=off
  wires:
  Msg/1 -> CANUnPackMessage4/2
  ID/1 -> CANUnPackMessage4/1
  CANUnPackMessage4/1 -> CAN Unpack/1
  CAN Unpack/2 -> MeaModule2/1
  CAN Unpack/3 -> IMU_Ay_Valid/1
  CAN Unpack/4 -> MeaModule4/1
  CAN Unpack/5 -> IMU_DTC/1
  CAN Unpack/7 -> MeaModule3/1
  CAN Unpack/6 -> IMU_Yaw_Valid/1
  CAN Unpack/1 -> IMU_Ax_Valid/1
  MeaModule2/1 -> IMU_Ax_Value/1
  MeaModule3/1 -> IMU_Yaw_Value/1
  MeaModule4/1 -> IMU_Ay_Value/1

== system VehCtrlMdel240926_2018b_amkspdlimit/Input/StrSnis_Receive/StrWhSnis_state/IMU_state ==
  ID : Inport
  Msg : Inport  Port=2
  Enable : EnablePort
  CAN Unpack : canmsglib/CAN Unpack  Commented=on  CANdbFile=d:\Users\YJR\Desktop\DBC\SWAS_3.dbc  MsgList=(none)  MsgName=PPEI_Steering_Wheel_Angle  MsgIDType=Standard (11-bit identifier)  MsgIdentifier=330  MsgLength=8  SignalInfo={'SAS_CheckSum','36','4','LE','unsigned','Standard','0','1','0','-Inf','Inf';'SAS_MassageCounter','32','4','LE','unsigned','Standard','0','1','0','0','15';'SAS_TrimmingFlag','26','1','LE','unsigned','Standard','0','1','0','0','255';'StrWhAng','8','16','BE','unsigned','Standard','0','1','0','0','65535';'StrWhAngV','16','8','LE','unsigned','Standard','0','1','0','0','1';'StrWhlAngSenCalFlag','25','1','LE','unsigned','Standard','0','1','0','0','3';'StrngWhlAngSnsrFailFlag','24','1','LE','unsigned','Standard','0','1','0','0','1'}  IDPort=off  TimestampPort=off  ErrorPort=off  RemotePort=off  LengthPort=off  StatusPort=off  ApplyMinMax=off
      settings: SourceProductName=Simulink Real-Time  SourceProductBaseCode=XP  DataFormat=CANdb specified signals
  CAN Unpack1 : canmsglib/CAN Unpack  CANdbFile=d:\Users\YJR\Desktop\DBC\SWAS.dbc  MsgList=PPEI_Steering_Wheel_Angle  MsgName=PPEI_Steering_Wheel_Angle  MsgIDType=Standard (11-bit identifier)  MsgIdentifier=330  MsgLength=8  SignalInfo={'StWhlAngAliveRollCnt','0','8','BE','unsigned','Standard','0','1','0','0','63';'StrWhAng','32','16','BE','unsigned','Standard','0','0.1','-779.3','-779.3','5774.2';'StrWhAngV','16','8','BE','unsigned','Standard','0','1','0','0','255'}  IDPort=off  TimestampPort=off  ErrorPort=off  RemotePort=off  LengthPort=off  StatusPort=off  ApplyMinMax=off
      settings: SourceProductName=Simulink Real-Time  SourceProductBaseCode=XP  DataFormat=CANdb specified signals
  CANUnPackMessage4 : ec5744lib/RapidECU_U3/04CANCommunication/CANUnPackMessage  datalength=8  canmessagetype=Standard(11-bit ID)  sampletime=-1
      settings: SourceProductName=ECUCoder for MPC5744
  MeaModule1 : ec5744lib/RapidECU_U3/07Calibration/MeaModule  signal=StrWhlAngAliveRollCnt
      settings: SourceProductName=ECUCoder for MPC5744
  MeaModule2 : ec5744lib/RapidECU_U3/07Calibration/MeaModule  signal=StrWhlAng
      settings: SourceProductName=ECUCoder for MPC5744
  MeaModule3 : ec5744lib/RapidECU_U3/07Calibration/MeaModule  signal=StrWhlAngV
      settings: SourceProductName=ECUCoder for MPC5744
  StrWhlAng : Outport  VectorParamsAs1DForOutWhenUnconnected=off
  StrWhlAngV : Outport  Port=2  VectorParamsAs1DForOutWhenUnconnected=off
  StrWhlAngAliveRollCnt : Outport  Port=3  VectorParamsAs1DForOutWhenUnconnected=off
  wires:
  Msg/1 -> CANUnPackMessage4/2
  ID/1 -> CANUnPackMessage4/1
  CANUnPackMessage4/1 -> CAN Unpack1/1
  CAN Unpack1/1 -> MeaModule1/1
  CAN Unpack1/2 -> MeaModule2/1
  CAN Unpack1/3 -> MeaModule3/1
  MeaModule1/1 -> StrWhlAngAliveRollCnt/1
  MeaModule2/1 -> StrWhlAng/1
  MeaModule3/1 -> StrWhlAngV/1

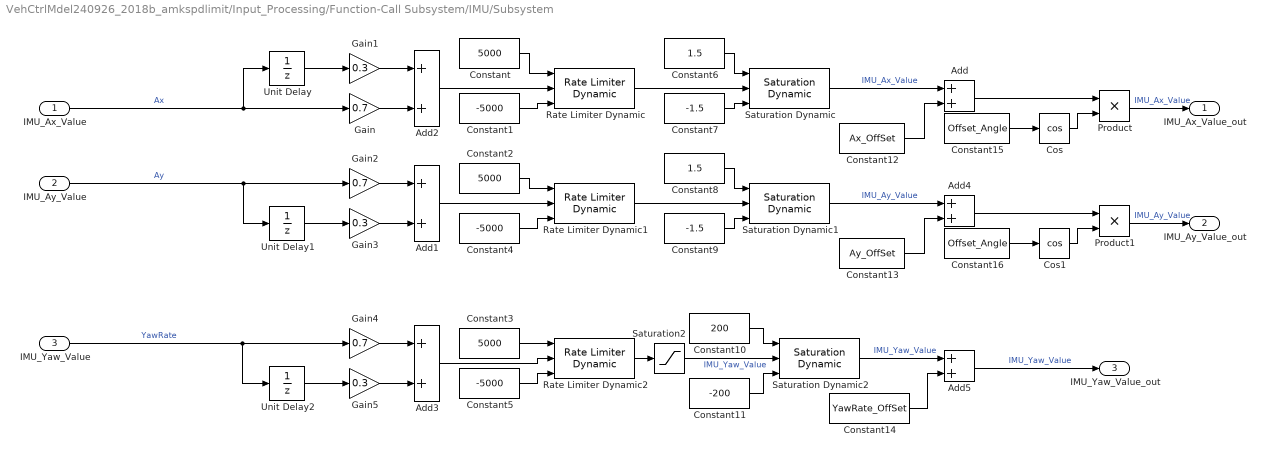
== system VehCtrlMdel240926_2018b_amkspdlimit/Input_Processing/Function-Call Subsystem/IMU/Subsystem ==
  IMU_Ax_Value : Inport
  IMU_Ay_Value : Inport  Port=2
  IMU_Yaw_Value : Inport  Port=3
  Add{,1..5} (6 alike) : Sum
  Constant : Constant  Value=5000
  Constant1 : Constant  Value=-5000
  Constant10 : Constant  Value=200  SampleTime=-1
  Constant11 : Constant  Value=-200  SampleTime=-1
  Constant12 : Constant  Value=Ax_OffSet
  Constant13 : Constant  Value=Ay_OffSet
  Constant14 : Constant  Value=YawRate_OffSet
  Constant15 : Constant  Value=Offset_Angle
  Constant16 : Constant  Value=Offset_Angle
  Constant2 : Constant  Value=5000
  Constant3 : Constant  Value=5000
  Constant4 : Constant  Value=-5000
  Constant5 : Constant  Value=-5000
  Constant6 : Constant  Value=1.5  SampleTime=-1
  Constant7 : Constant  Value=-1.5  SampleTime=-1
  Constant8 : Constant  Value=1.5  SampleTime=-1
  Constant9 : Constant  Value=-1.5  SampleTime=-1
  Cos : Trigonometry  Operator=cos
  Cos1 : Trigonometry  Operator=cos
  Gain : Gain  Gain=0.7
  Gain1 : Gain  Gain=0.3
  Gain2 : Gain  Gain=0.7
  Gain3 : Gain  Gain=0.3
  Gain4 : Gain  Gain=0.7
  Gain5 : Gain  Gain=0.3
  Product : Product
  Product1 : Product
  Rate Limiter Dynamic : simulink/Discontinuities/Rate Limiter Dynamic
      settings: SourceProductName=Simulink
  Rate Limiter Dynamic1 : simulink/Discontinuities/Rate Limiter Dynamic
      settings: SourceProductName=Simulink
  Rate Limiter Dynamic2 : simulink/Discontinuities/Rate Limiter Dynamic
      settings: SourceProductName=Simulink
  Saturation Dynamic : simulink/Discontinuities/Saturation Dynamic  OutMin=[]  OutMax=[]  OutDataTypeStr=Inherit: Same as second input  OutDataType=fixdt(1, 16)  OutScaling=2^-10  DoSatur=off
  Saturation Dynamic1 : simulink/Discontinuities/Saturation Dynamic  OutMin=[]  OutMax=[]  OutDataTypeStr=Inherit: Same as second input  OutDataType=fixdt(1, 16)  OutScaling=2^-10  DoSatur=off
  Saturation Dynamic2 : simulink/Discontinuities/Saturation Dynamic  OutMin=[]  OutMax=[]  OutDataTypeStr=Inherit: Same as second input  OutDataType=fixdt(1, 16)  OutScaling=2^-10  DoSatur=off
  Saturation2 : Saturate  UpperLimit=180  LowerLimit=-180
  Unit Delay : UnitDelay  SampleTime=-1  HasFrameUpgradeWarning=on
  Unit Delay1 : UnitDelay  SampleTime=-1  HasFrameUpgradeWarning=on
  Unit Delay2 : UnitDelay  SampleTime=-1  HasFrameUpgradeWarning=on
  IMU_Ax_Value_out : Outport  VectorParamsAs1DForOutWhenUnconnected=off
  IMU_Ay_Value_out : Outport  Port=2  VectorParamsAs1DForOutWhenUnconnected=off
  IMU_Yaw_Value_out : Outport  Port=3  VectorParamsAs1DForOutWhenUnconnected=off
  wires:
  IMU_Ay_Value/1 -> Unit Delay1/1, Gain2/1  "Ay"
  Unit Delay/1 -> Gain1/1
  Gain/1 -> Add2/2
  Constant2/1 -> Rate Limiter Dynamic1/1
  Constant/1 -> Rate Limiter Dynamic/1
  Add2/1 -> Rate Limiter Dynamic/2
  Gain2/1 -> Add1/1
  IMU_Yaw_Value/1 -> Gain4/1, Unit Delay2/1  "YawRate"
  Gain1/1 -> Add2/1
  Gain5/1 -> Add3/2
  IMU_Ax_Value/1 -> Gain/1, Unit Delay/1  "Ax"
  Constant11/1 -> Saturation Dynamic2/3
  Add1/1 -> Rate Limiter Dynamic1/2
  Unit Delay1/1 -> Gain3/1
  Constant8/1 -> Saturation Dynamic1/1
  Add3/1 -> Rate Limiter Dynamic2/2
  Constant4/1 -> Rate Limiter Dynamic1/3
  Rate Limiter Dynamic1/1 -> Saturation Dynamic1/2
  Constant1/1 -> Rate Limiter Dynamic/3
  Gain4/1 -> Add3/1
  Constant7/1 -> Saturation Dynamic/3
  Constant3/1 -> Rate Limiter Dynamic2/1
  Product/1 -> IMU_Ax_Value_out/1  "IMU_Ax_Value"
  Constant9/1 -> Saturation Dynamic1/3
  Add5/1 -> IMU_Yaw_Value_out/1  "IMU_Yaw_Value"
  Rate Limiter Dynamic2/1 -> Saturation2/1
  Saturation2/1 -> Saturation Dynamic2/2  "IMU_Yaw_Value"
  Constant10/1 -> Saturation Dynamic2/1
  Constant5/1 -> Rate Limiter Dynamic2/3
  Rate Limiter Dynamic/1 -> Saturation Dynamic/2
  Gain3/1 -> Add1/2
  Product1/1 -> IMU_Ay_Value_out/1  "IMU_Ay_Value"
  Constant6/1 -> Saturation Dynamic/1
  Unit Delay2/1 -> Gain5/1
  Saturation Dynamic/1 -> Add/1  "IMU_Ax_Value"
  Constant12/1 -> Add/2
  Saturation Dynamic1/1 -> Add4/1  "IMU_Ay_Value"
  Constant13/1 -> Add4/2
  Saturation Dynamic2/1 -> Add5/1  "IMU_Yaw_Value"
  Constant14/1 -> Add5/2
  Add/1 -> Product/1
  Cos/1 -> Product/2
  Constant15/1 -> Cos/1
  Constant16/1 -> Cos1/1
  Cos1/1 -> Product1/2
  Add4/1 -> Product1/1

== system VehCtrlMdel240926_2018b_amkspdlimit/Input_Processing/Subsystem/WhlSlpageJudgment/加速度差判断 ==
  note: 输出“1”代表判定有效
  <VxFL_mps> : Inport
  <VxFR_mps> : Inport  Port=2
  <VxRL_mps> : Inport  Port=3
  <VxRR_mps> : Inport  Port=4
  IMU_Ax_mpss : Inport  Port=5
  Abs{,1..3} (4 alike) : Abs
  Add{,1..3} (4 alike) : Sum  Inputs=+-
  Add{4..7} (4 alike) : Sum  Inputs=-+
  Compare To Constant{,1..3} (4 alike) : simulink/Logic and Bit Operations/Compare To Constant  relop=<=  const=thr2  OutDataTypeStr=boolean
  Divide{,1..3} (4 alike) : Product  Inputs=*/
  Filter : Subsystem
  Filter1 : Subsystem
  Filter2 : Subsystem
  Filter3 : Subsystem
  Unit Delay{,1..3} (4 alike) : UnitDelay  SampleTime=-1  HasFrameUpgradeWarning=on
  steptime{,1..3} (4 alike) : Constant  Value=single(0.01)
  y : Outport
  y1 : Outport  Port=2
  y2 : Outport  Port=3
  y3 : Outport  Port=4
  wires:
  Compare To Constant/1 -> y/1
  Compare To Constant2/1 -> y2/1
  Abs2/1 -> Compare To Constant2/1
  Add1/1 -> Abs1/1
  Abs/1 -> Compare To Constant/1
  [IMU_Ax_mpss] -> Add3/2
  [IMU_Ax_mpss] -> Add2/2
  [IMU_Ax_mpss] -> Add/2
  Abs3/1 -> Compare To Constant3/1
  Compare To Constant3/1 -> y3/1
  Compare To Constant1/1 -> y1/1
  [IMU_Ax_mpss] -> Add1/2
  Add/1 -> Abs/1
  Add3/1 -> Abs3/1
  Abs1/1 -> Compare To Constant1/1
  Add2/1 -> Abs2/1
  <VxFL_mps>/1 -> Add4/2, Unit Delay/1
  Unit Delay/1 -> Add4/1
  Add4/1 -> Divide/1
  steptime/1 -> Divide/2
  Divide/1 -> Filter/1(In)
  IMU_Ax_mpss/1 -> [IMU_Ax_mpss]
  steptime1/1 -> Divide1/2
  Add5/1 -> Divide1/1
  Unit Delay1/1 -> Add5/1
  <VxFR_mps>/1 -> Unit Delay1/1, Add5/2
  Divide1/1 -> Filter1/1(In)
  steptime2/1 -> Divide2/2
  Add6/1 -> Divide2/1
  Unit Delay2/1 -> Add6/1
  <VxRL_mps>/1 -> Unit Delay2/1, Add6/2
  Divide2/1 -> Filter2/1(In)
  steptime3/1 -> Divide3/2
  Add7/1 -> Divide3/1
  Unit Delay3/1 -> Add7/1
  <VxRR_mps>/1 -> Unit Delay3/1, Add7/2
  Divide3/1 -> Filter3/1(In)
  Filter/1(Out) -> Add/1
  Filter1/1(Out) -> Add1/1
  Filter2/1(Out) -> Add2/1
  Filter3/1(Out) -> Add3/1

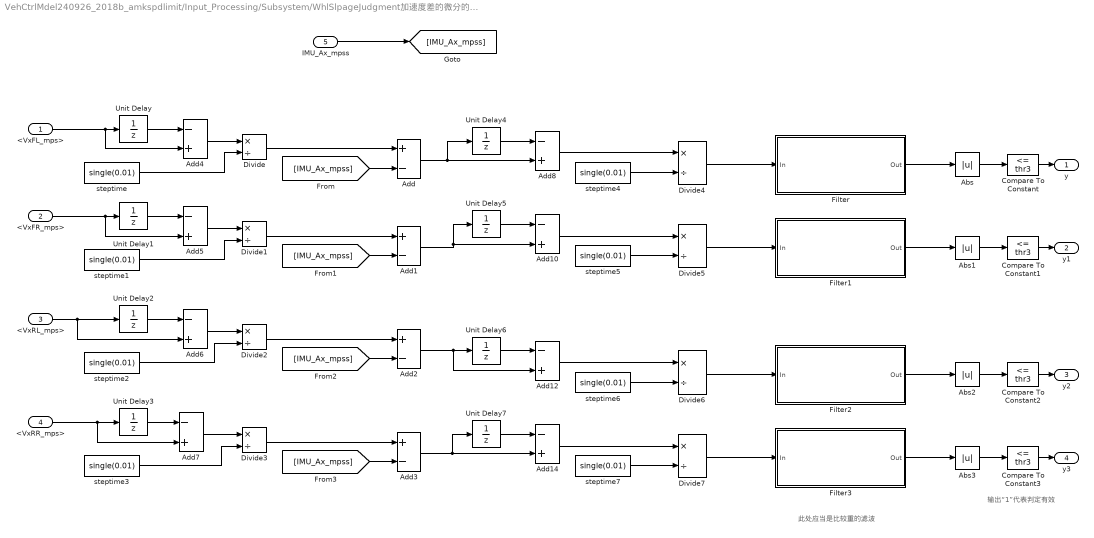
== system VehCtrlMdel240926_2018b_amkspdlimit/Input_Processing/Subsystem/WhlSlpageJudgment/加速度差的微分的判断 ==
  note: 此处应当是比较重的滤波
  note: 输出“1”代表判定有效
  <VxFL_mps> : Inport
  <VxFR_mps> : Inport  Port=2
  <VxRL_mps> : Inport  Port=3
  <VxRR_mps> : Inport  Port=4
  IMU_Ax_mpss : Inport  Port=5
  Abs{,1..3} (4 alike) : Abs
  Add{,1..3} (4 alike) : Sum  Inputs=+-
  Add{4..8,10,12,14} (8 alike) : Sum  Inputs=-+
  Compare To Constant{,1..3} (4 alike) : simulink/Logic and Bit Operations/Compare To Constant  relop=<=  const=thr3  OutDataTypeStr=boolean
  Divide{,1..7} (8 alike) : Product  Inputs=*/
  Filter : Subsystem
  Filter1 : Subsystem
  Filter2 : Subsystem
  Filter3 : Subsystem
  Unit Delay{,1..7} (8 alike) : UnitDelay  SampleTime=-1  HasFrameUpgradeWarning=on
  steptime{,1..7} (8 alike) : Constant  Value=single(0.01)
  y : Outport
  y1 : Outport  Port=2
  y2 : Outport  Port=3
  y3 : Outport  Port=4
  wires:
  Divide3/1 -> Add3/1
  <VxRR_mps>/1 -> Add7/2, Unit Delay3/1
  Unit Delay3/1 -> Add7/1
  Add7/1 -> Divide3/1
  steptime3/1 -> Divide3/2
  Divide2/1 -> Add2/1
  <VxRL_mps>/1 -> Add6/2, Unit Delay2/1
  Unit Delay2/1 -> Add6/1
  Add6/1 -> Divide2/1
  steptime2/1 -> Divide2/2
  Divide1/1 -> Add1/1
  <VxFR_mps>/1 -> Add5/2, Unit Delay1/1
  Unit Delay1/1 -> Add5/1
  Add5/1 -> Divide1/1
  steptime1/1 -> Divide1/2
  IMU_Ax_mpss/1 -> [IMU_Ax_mpss]
  Divide/1 -> Add/1
  steptime/1 -> Divide/2
  Add4/1 -> Divide/1
  Unit Delay/1 -> Add4/1
  <VxFL_mps>/1 -> Unit Delay/1, Add4/2
  Abs1/1 -> Compare To Constant1/1
  [IMU_Ax_mpss] -> Add1/2
  Compare To Constant1/1 -> y1/1
  Compare To Constant3/1 -> y3/1
  Abs3/1 -> Compare To Constant3/1
  [IMU_Ax_mpss] -> Add/2
  [IMU_Ax_mpss] -> Add2/2
  [IMU_Ax_mpss] -> Add3/2
  Abs/1 -> Compare To Constant/1
  Abs2/1 -> Compare To Constant2/1
  Compare To Constant2/1 -> y2/1
  Compare To Constant/1 -> y/1
  Add/1 -> Add8/2, Unit Delay4/1
  Unit Delay4/1 -> Add8/1
  Add8/1 -> Divide4/1
  steptime4/1 -> Divide4/2
  Divide4/1 -> Filter/1(In)
  steptime5/1 -> Divide5/2
  Add10/1 -> Divide5/1
  Unit Delay5/1 -> Add10/1
  Add1/1 -> Unit Delay5/1, Add10/2
  Divide5/1 -> Filter1/1(In)
  Divide6/1 -> Filter2/1(In)
  Add2/1 -> Add12/2, Unit Delay6/1
  Add12/1 -> Divide6/1
  steptime6/1 -> Divide6/2
  Unit Delay6/1 -> Add12/1
  steptime7/1 -> Divide7/2
  Add14/1 -> Divide7/1
  Add3/1 -> Unit Delay7/1, Add14/2
  Unit Delay7/1 -> Add14/1
  Divide7/1 -> Filter3/1(In)
  Filter/1(Out) -> Abs/1
  Filter1/1(Out) -> Abs1/1
  Filter2/1(Out) -> Abs2/1
  Filter3/1(Out) -> Abs3/1

== system VehCtrlMdel240926_2018b_amkspdlimit/Input_Processing/Subsystem/WhlSlpageJudgment/速差判断 ==
  note: 输出“1”代表判定有效
  <VxFL_mps> : Inport
  <VxFR_mps> : Inport  Port=2
  <VxRL_mps> : Inport  Port=3
  <VxRR_mps> : Inport  Port=4
  VehSpd_mps : Inport  Port=5
  In6 : Inport  Port=6
  AND{,1..3} (4 alike) : Logic  AllPortsSameDT=off  OutDataTypeStr=boolean
  Abs{,1..3} (4 alike) : Abs
  Add{,1..3} (4 alike) : Sum  Inputs=+-
  Bus Selector1 : BusSelector  OutputSignals=WhlSpdii_mps.WhlSpdRL_Valid,WhlSpdii_mps.WhlSpdRR_Valid,WhlSpdii_mps.WhlSpdFR_Valid,WhlSpdii_mps.WhlSpdFL_Valid
  Compare To Constant{,1..3} (4 alike) : simulink/Logic and Bit Operations/Compare To Constant  relop=<=  const=thr1  OutDataTypeStr=boolean
  y : Outport
  y1 : Outport  Port=2
  y2 : Outport  Port=3
  y3 : Outport  Port=4
  wires:
  Add2/1 -> Abs2/1
  Abs1/1 -> Compare To Constant1/1
  <VxRR_mps>/1 -> Add3/1
  Add3/1 -> Abs3/1
  Add/1 -> Abs/1
  [VehSpd_mps] -> Add1/2
  <VxRL_mps>/1 -> Add2/1
  <VxFR_mps>/1 -> Add1/1
  Compare To Constant1/1 -> AND2/1
  Compare To Constant3/1 -> AND1/1
  Abs3/1 -> Compare To Constant3/1
  [VehSpd_mps] -> Add/2
  [VehSpd_mps] -> Add2/2
  [VehSpd_mps] -> Add3/2
  Abs/1 -> Compare To Constant/1
  Add1/1 -> Abs1/1
  Abs2/1 -> Compare To Constant2/1
  <VxFL_mps>/1 -> Add/1
  Compare To Constant2/1 -> AND/1
  Compare To Constant/1 -> AND3/1
  VehSpd_mps/1 -> [VehSpd_mps]
  In6/1 -> Bus Selector1/1
  Bus Selector1/1 -> AND/2  "<WhlSpdRL_Valid>"
  Bus Selector1/2 -> AND1/2  "<WhlSpdRR_Valid>"
  Bus Selector1/3 -> AND2/2  "<WhlSpdFR_Valid>"
  Bus Selector1/4 -> AND3/2  "<WhlSpdFL_Valid>"
  AND3/1 -> y/1
  AND2/1 -> y1/1
  AND1/1 -> y3/1
  AND/1 -> y2/1

== system VehCtrlMdel240926_2018b_amkspdlimit/Input_Processing/Subsystem/WhlSpdSelect/Filter ==
  In : Inport
  Add : Sum
  Constant : Constant  Value=single(0)
  Constant1 : Constant  Value=single(100)
  Constant2 : Constant  Value=single(15)
  Constant3 : Constant  Value=single(-15)
  Gain : Gain  Gain=0
  Gain1 : Gain
  Rate Limiter Dynamic : simulink/Discontinuities/Rate Limiter Dynamic
      settings: SourceProductName=Simulink
  Saturation Dynamic : simulink/Discontinuities/Saturation Dynamic  OutMin=[]  OutMax=[]  OutDataTypeStr=Inherit: Same as second input  OutDataType=fixdt(1, 16)  OutScaling=2^-10  DoSatur=off
  Unit Delay : UnitDelay  SampleTime=-1  HasFrameUpgradeWarning=on
  VehVxEst_mps : Outport
  wires:
  In/1 -> Saturation Dynamic/2
  Saturation Dynamic/1 -> Rate Limiter Dynamic/2
  Constant1/1 -> Saturation Dynamic/1
  Constant/1 -> Saturation Dynamic/3
  Unit Delay/1 -> Gain/1
  Gain/1 -> Add/1
  Gain1/1 -> Add/2
  Rate Limiter Dynamic/1 -> Gain1/1, Unit Delay/1
  Add/1 -> VehVxEst_mps/1
  Constant2/1 -> Rate Limiter Dynamic/1
  Constant3/1 -> Rate Limiter Dynamic/3

== system VehCtrlMdel240926_2018b_amkspdlimit/Input_Processing/Subsystem/WhlSpdSelect/Subsystem ==
  <VxFL_mps> : Inport
  <VxFR_mps> : Inport  Port=2
  <VxRL_mps> : Inport  Port=3
  <VxRR_mps> : Inport  Port=4
  Add3 : Sum  Inputs=++++
  Add4 : Sum  Inputs=+--
  Gain1 : Gain  Gain=1/2
  Min3 : MinMax  Function=max  Inputs=4
  Min4 : MinMax  Inputs=4
  Subsystem : Subsystem  Commented=on
  MiddleWhlSpd_mps : Outport
  wires:
  Add4/1 -> Gain1/1
  Add3/1 -> Add4/1
  Min3/1 -> Add4/3
  <VxRR_mps>/1 -> Min3/4, Add3/1, Min4/4
  <VxRL_mps>/1 -> Min3/3, Min4/3, Add3/2
  <VxFR_mps>/1 -> Min4/2, Min3/2, Add3/3
  Min4/1 -> Add4/2
  <VxFL_mps>/1 -> Add3/4, Min4/1, Min3/1
  Gain1/1 -> MiddleWhlSpd_mps/1  "MaxWhlSpd_mps"
